simulink model "sound_agg_fal"  (Simulink 10.1)
settings: Solver=FixedStepAuto  StartTime=0.0  StopTime=60  FixedStep=fixedStep  MaxStep=0.2  RelTol=1e-3
values from neighbouring files (symbols this model uses):
  configSoundSource = [1 58]    [garbageDisposalInit.m]
  disSoundSource = disGarbageDisposal    [garbageDisposalInit.m]
undefined symbols (not defined in the file or in its folder): configSoundSource2, configSoundSource3, disSoundSource2, disSoundSource3
settings Model: Creator=lixuansong  LastModifiedBy=ozgurozmen
settings DataIOCC: SaveOutput=off  SignalLogging=off  DSMLogging=off  SaveTime=off
settings OptimizationCC: LifeSpan=auto
settings DebuggingCC: UnderspecifiedInitializationDetection=Simplified  MergeDetectMultiDrivingBlocksExec=error  SFUnexpectedBacktrackingDiag=error  SFNoUnconditionalDefaultTransitionDiag=error  SFExecutionAtInitializationDiag=warning  ArithmeticOperatorsInVariantConditions=error
settings HardwareCC: ProdBitPerPointer=64  ProdBitPerSizeT=64  ProdBitPerPtrDiffT=64  ProdLargestAtomicFloat=Float  ProdIntDivRoundTo=Zero  ProdEndianess=LittleEndian  ProdWordSize=64  ProdHWDeviceType=Intel->x86-64 (Windows64)
settings ModelReferenceCC: PropagateSignalLabelsOutOfModel=on
settings SFSimCC: SimUseLocalCustomCode=on  CustomCodeUndefinedFunction=FilterOut
settings RTWCC: RTWUseLocalCustomCode=on
settings CodeAppCC: StateflowObjectComments=off
settings GRTTargetCC: TargetLangStandard=C99 (ISO)  CombineOutputUpdateFcns=on  GRTInterface=off
settings ConfigComp: CovMetricSettings=dwe  CovHtmlReporting=off  CovSaveCumulativeToWorkspaceVar=off  CovSaveSingleToWorkspaceVar=off  CovExternalEMLEnable=on

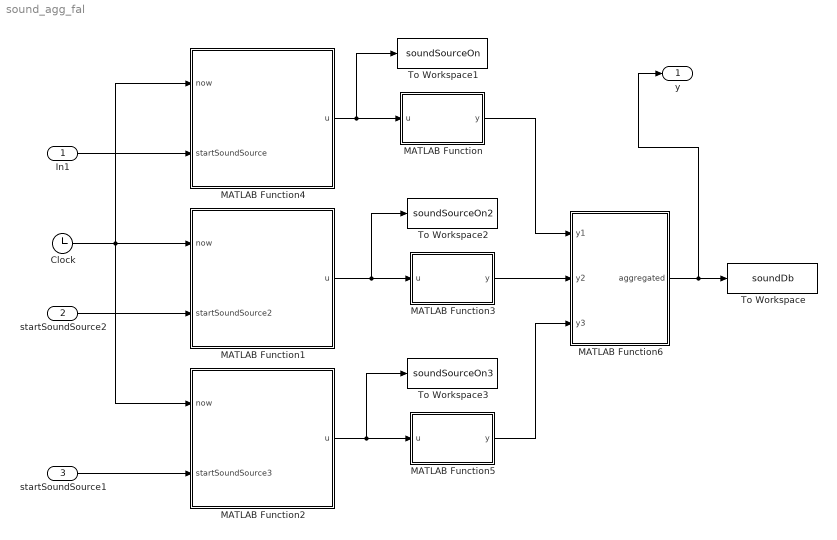
== system sound_agg_fal ==
  In1 : Inport
  startSoundSource2 : Inport  Port=2
  startSoundSource1 : Inport  Port=3
  Clock : Clock
  MATLAB Function : MATLAB Function  TreatAsAtomicUnit=on
  MATLAB Function1 : MATLAB Function  TreatAsAtomicUnit=on
  MATLAB Function2 : MATLAB Function  TreatAsAtomicUnit=on
  MATLAB Function3 : MATLAB Function  TreatAsAtomicUnit=on
  MATLAB Function4 : MATLAB Function  TreatAsAtomicUnit=on
  MATLAB Function5 : MATLAB Function  TreatAsAtomicUnit=on
  MATLAB Function6 : MATLAB Function  TreatAsAtomicUnit=on
  To Workspace : ToWorkspace  VariableName=soundDb  SampleTime=-1
  To Workspace1 : ToWorkspace  VariableName=soundSourceOn  SampleTime=-1
  To Workspace2 : ToWorkspace  VariableName=soundSourceOn2  SampleTime=-1
  To Workspace3 : ToWorkspace  VariableName=soundSourceOn3  SampleTime=-1
  y : Outport
  wires:
  MATLAB Function4/1(u) -> To Workspace1/1, MATLAB Function/1(u)
  In1/1 -> MATLAB Function4/2(startSoundSource)
  startSoundSource2/1 -> MATLAB Function1/2(startSoundSource2)
  startSoundSource1/1 -> MATLAB Function2/2(startSoundSource3)
  Clock/1 -> MATLAB Function2/1(now), MATLAB Function1/1(now), MATLAB Function4/1(now)
  MATLAB Function1/1(u) -> To Workspace2/1, MATLAB Function3/1(u)
  MATLAB Function2/1(u) -> To Workspace3/1, MATLAB Function5/1(u)
  MATLAB Function/1(y) -> MATLAB Function6/1(y1)
  MATLAB Function3/1(y) -> MATLAB Function6/2(y2)
  MATLAB Function5/1(y) -> MATLAB Function6/3(y3)
  MATLAB Function6/1(aggregated) -> y/1, To Workspace/1

== matlab function MATLAB Function1 ==
  data: u output double; now input double; timeSoundSource2 parameter double; startSoundSource2 input double
function u = controlSoundSource2(now,timeSoundSource2, startSoundSource2)
if now>=startSoundSource2 && now<=startSoundSource2+timeSoundSource2
    u=1;
else
    u=0;
end

== matlab function MATLAB Function ==
  data: u input double; y output double; disSoundSource parameter double; configSoundSource parameter double
function y = calSound(u, disSoundSource,configSoundSource)

dis0=configSoundSource(1);%distance in configuration
db0=configSoundSource(2);%db in configuration

if u==1
    y=db0-log2(disSoundSource/dis0)*6;
else
    y=0;
end

== matlab function MATLAB Function2 ==
  data: u output double; now input double; timeSoundSource3 parameter double; startSoundSource3 input double
function u = controlSoundSource3(now,timeSoundSource3, startSoundSource3)
if now>=startSoundSource3 && now<=startSoundSource3+timeSoundSource3
    u=1;
else
    u=0;
end

== matlab function MATLAB Function3 ==
  data: u input double; y output double; disSoundSource2 parameter double; configSoundSource2 parameter double
function y = calSound(u, disSoundSource2,configSoundSource2)

dis0=configSoundSource2(1);%distance in configuration
db0=configSoundSource2(2);%db in configuration

if u==1
    y=db0-log2(disSoundSource2/dis0)*6;
else
    y=0;
end

== matlab function MATLAB Function4 ==
  data: u output double; now input double; timeSoundSource parameter double; startSoundSource input double
function u = controlSoundSource(now,timeSoundSource, startSoundSource)
if now>=startSoundSource && now<=startSoundSource+timeSoundSource
    u=1;
else
    u=0;
end

== matlab function MATLAB Function5 ==
  data: u input double; y output double; disSoundSource3 parameter double; configSoundSource3 parameter double
function y = calSound(u, disSoundSource3,configSoundSource3)

dis0=configSoundSource3(1);%distance in configuration
db0=configSoundSource3(2);%db in configuration

if u==1
    y=db0-log2(disSoundSource3/dis0)*6;
else
    y=0;
end

== matlab function MATLAB Function6 ==
  data: y1 input double; aggregated output double; y2 input double; y3 input double
function aggregated = AggSound(y1, y2, y3)

aggregated = 10*log10(10^(y1/10) + 10^(y2/10) + 10^(y3/10));



end
